simulink model "Exp4_PartA_19EE10039_1"  (R2021a)
settings: Solver=VariableStepAuto  StartTime=0.0  StopTime=0.04  RelTol=1e-3
libraries: spsGroundLib x2, spsMonostableLib x2, spsVoltageMeasurementLib x2, spsACVoltageSourceLib x1, spsDCVoltageSourceLib x1, simulink_extras x1, spsLinearTransformerLib x1, spspowerguiLib x1
settings Model: Creator=USER  LastModifiedBy=mansi

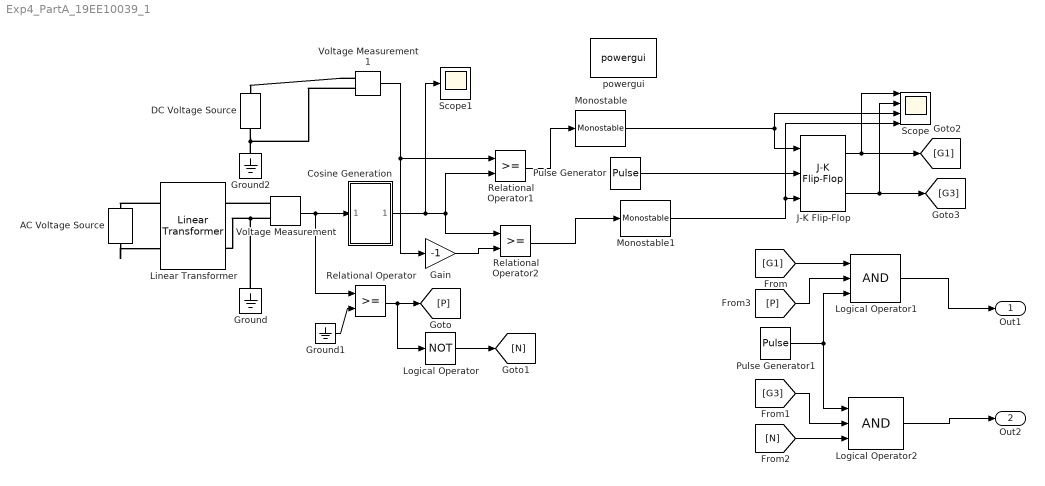
== system Exp4_PartA_19EE10039_1 ==
  AC Voltage Source : spsACVoltageSourceLib/AC Voltage Source  Amplitude=230*sqrt(2)  Phase=0  Frequency=50  SampleTime=0  Measurements=None  BusType=swing  Pref=10e3  Qref=0  Qmin=-inf  Qmax=+inf
  Cosine Generation : Subsystem
  DC Voltage Source : spsDCVoltageSourceLib/DC Voltage Source  Amplitude=4.015  Measurements=None
  Gain : Gain  Gain=-1
  Ground : spsGroundLib/Ground  LConnTagsString=a
  Ground1 : Ground
  Ground2 : spsGroundLib/Ground  LConnTagsString=a
  J-K Flip-Flop : simulink_extras/Flip Flops/J-K Flip-Flop  initial_condition=0
  Linear Transformer : spsLinearTransformerLib/Linear Transformer  UNITS=SI  NominalPower=[4 50]  winding1=[230 6.9 7.1e-3]  winding2=[3.605 1.7e-3 2.1e-6]  ThreeWindings=off  winding3=[3.15e+05 315.06 0.10641]  RmLm=[600 1.145]  Measurements=None  DataType=on
  Logical Operator : Logic  Operator=NOT  Inputs=1  IconShape=distinctive  AllPortsSameDT=off  OutDataTypeStr=boolean
  Logical Operator1 : Logic  Inputs=3  IconShape=distinctive  AllPortsSameDT=off  OutDataTypeStr=boolean
  Logical Operator2 : Logic  Inputs=3  IconShape=distinctive  AllPortsSameDT=off  OutDataTypeStr=boolean
  Monostable : spsMonostableLib/Monostable  EdgeDetect=Rising  PulseDuration=1e-5  ic=0  Ts=0
      settings: SourceProductBaseCode=PS
  Monostable1 : spsMonostableLib/Monostable  EdgeDetect=Rising  PulseDuration=1e-5  ic=0  Ts=0
      settings: SourceProductBaseCode=PS
  Pulse Generator : DiscretePulseGenerator  PulseType=Time based  Period=2e-6  PulseWidth=50
  Pulse Generator1 : DiscretePulseGenerator  PulseType=Time based  Period=40e-6  PulseWidth=50
  Relational Operator : RelationalOperator  OutDataTypeStr=boolean  RndMeth=Simplest
  Relational Operator1 : RelationalOperator  OutDataTypeStr=boolean  RndMeth=Simplest
  Relational Operator2 : RelationalOperator  OutDataTypeStr=boolean  RndMeth=Simplest
  Scope : Scope  NumInputPorts=4
  Scope1 : Scope
  Voltage Measurement : spsVoltageMeasurementLib/Voltage Measurement  PhasorSimulation=off  OutputType=Complex  PSBequivalent=0
  Voltage Measurement1 : spsVoltageMeasurementLib/Voltage Measurement  PhasorSimulation=off  OutputType=Complex  PSBequivalent=0
  powergui : spspowerguiLib/powergui  Priority=1  SimulationMode=Discrete  SampleTime=1e-6  frequency=60  Iterations=50  frequencyindice=0  Pbase=100e6  ErrMax=1e-4  UnitsV=kV  UnitsW=MW  buscounter=0  FunctionMessages=off  echomessages=off  EnableUseOfTLC=off  CurrentSourceSwitches=off  DisableSnubberDevices=off  DisableRonSwitches=off  DisableVfSwitches=off  DisplayEquations=off  AutomaticDiscreteSolvers=off  SolverType=Tustin/Backward Euler (TBE)  Interpol=off  ExternalGateDelay=off  methode=off  Ts=10  x0status=blocks  SPID=off  SwTol=0  HookPort=off  NonlinearTolerance=1e-4  nMaxIteration=100  ContinueOnMaxIteration=off  RestoreLinks=warning  ResistiveCurrentMeasurement=off  Frange=[0:2:500]  Ylog=off  Xlog=on  ShowGrid=off  save=off  variable=ZData  structure=ScopeData10  ZoomFFT=off  StartTime=0.124  cycles=2  DisplayStyle=2  fundamental=50  FreqAxis=on  MaxFrequency=5000  frequencyindicesteady=1  RmsSteady=1  display=off
  Out1 : Outport
  Out2 : Outport  Port=2
  wires:
  [G1] -> Logical Operator1/1
  J-K Flip-Flop/2 -> Scope/2, [G3]
  Logical Operator2/1 -> Out2/1
  [P] -> Logical Operator1/2
  J-K Flip-Flop/1 -> Scope/1, [G1]
  Relational Operator2/1 -> Monostable1/1
  Voltage Measurement/1 -> Cosine Generation/1(In1), Relational Operator/1
  Logical Operator/1 -> [N]
  Gain/1 -> Relational Operator2/2
  [G3] -> Logical Operator2/2
  Monostable1/1 -> Scope/4, J-K Flip-Flop/3
  Ground1/1 -> Relational Operator/2
  Voltage Measurement1/1 -> Gain/1, Relational Operator1/1
  Pulse Generator1/1 -> Logical Operator2/1, Logical Operator1/3
  [N] -> Logical Operator2/3
  Logical Operator1/1 -> Out1/1
  Monostable/1 -> J-K Flip-Flop/1, Scope/3
  Pulse Generator/1 -> J-K Flip-Flop/2
  Relational Operator/1 -> Logical Operator/1, [P]
  Relational Operator1/1 -> Monostable/1
  Cosine Generation/1(Out1) -> Scope1/1, Relational Operator1/2, Relational Operator2/1
  connections:
  Voltage Measurement/LConn2 -- Ground/LConn1 -- Linear Transformer/RConn2
  Ground2/LConn1 -- Voltage Measurement1/LConn2 -- DC Voltage Source/LConn1
  Linear Transformer/LConn1 -- AC Voltage Source/RConn1
  Voltage Measurement/LConn1 -- Linear Transformer/RConn1
  Voltage Measurement1/LConn1 -- DC Voltage Source/RConn1
  AC Voltage Source/LConn1 -- Linear Transformer/LConn2

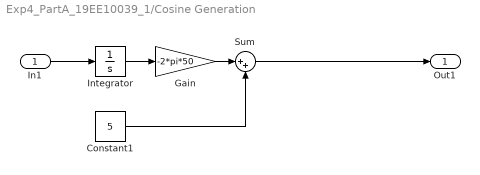
== system Exp4_PartA_19EE10039_1/Cosine Generation ==
  In1 : Inport
  Constant1 : Constant  Value=5
  Gain : Gain  Gain=-2*pi*50
  Integrator : Integrator
  Sum : Sum  Inputs=|++
  Out1 : Outport
  wires:
  Sum/1 -> Out1/1
  Constant1/1 -> Sum/2
  In1/1 -> Integrator/1
  Integrator/1 -> Gain/1
  Gain/1 -> Sum/1
